simulink model "sonusimulink"  (R2015a)
settings: Solver=ode23tb  StartTime=0.0  StopTime=2  MaxStep=10e-6  RelTol=1e-3
InitFcn:
  | fs=1000;
libraries: powerlib x26, simulink x2
settings Model: Creator=KASHIF  LastModifiedBy=NITIN
settings DataIOCC: SignalLoggingSaveFormat=ModelDataLogs
settings OptimizationCC: ExpressionDepthLimit=2147483647
settings DebuggingCC: UnderspecifiedInitializationDetection=Classic  MergeDetectMultiDrivingBlocksExec=none  SolverPrmCheckMsg=warning  FcnCallInpInsideContextMsg=UseLocalSettings  StateNameClashWarn=warning
settings GRTTargetCC: CombineOutputUpdateFcns=off  GRTInterface=on

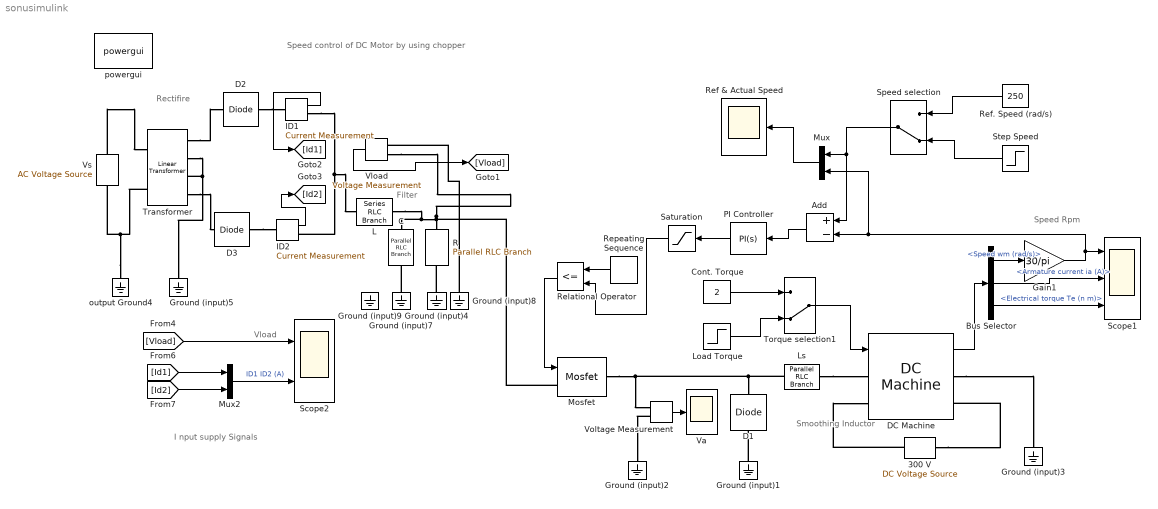
== system sonusimulink ==
  note: Speed control of DC Motor by using chopper
  note: Vload
  note: I nput supply Signals
  note: Rectifire
  note: Filter
  note: Speed Rpm
  note: Smoothing
      |  Inductor
  300 V : powerlib/Electrical Sources/DC Voltage Source  Description=source block  Amplitude=300  Measurements=None
      settings: AttributesFormatString=\n
  Add : Sum  Inputs=+-
  Bus Selector : BusSelector  OutputSignals=Speed wm (rad/s),Armature current ia (A),Electrical torque Te (n m)
  C : powerlib/Elements/Parallel RLC Branch  LConnTagsString=a  RConnTagsString=__new0  BranchType=C  Resistance=5  Inductance=1.0  SetiL0=off  InitialCurrent=0  Capacitance=500e-06  Setx0=off  InitialVoltage=0  Measurements=None
  Cont. Torque : Constant  Value=2
  D1 : powerlib/Power Electronics/Diode  Ron=0.05  Lon=0  Vf=0.7  IC=0  UseSnubber=off  Rs=Inf  Cs=0.1e-6  Measurements=off
  D2 : powerlib/Power Electronics/Diode  Ron=1e-3  Lon=0  Vf=0.7  IC=0  UseSnubber=off  Rs=1e6  Cs=inf  Measurements=off
  D3 : powerlib/Power Electronics/Diode  Ron=1e-3  Lon=0  Vf=0.7  IC=0  UseSnubber=off  Rs=1e6  Cs=inf  Measurements=off
  DC Machine : powerlib/Machines/DC Machine  PresetModel=01: 5HP 240V 1750RPM Field:300V  MechanicalLoad=Torque TL  FieldType=Wound  ShowDetailedParameters=on  MeasurementBus=off  RLa=[2.581 0.028]  RLf=[281.3 156]  Laf=0.9483  MachineConstant=Torque constant (N.m/A)  Ke=1.8  Kt=1.8  J=0.02215  Bm=0.002953  Tf=0.5161  w0=1  Ifinit=1  TsPowergui=0  TsBlock=-1
      settings: AttributesFormatString=\n
  Gain1 : Gain  Gain=30/pi
  Ground (input){1..5,7..9} (8 alike) : powerlib/Elements/Ground  LConnTagsString=a
  ID1 : powerlib/Measurements/Current Measurement  PhasorSimulation=off  OutputType=Complex  PSBequivalent=0
  ID2 : powerlib/Measurements/Current Measurement  PhasorSimulation=off  OutputType=Complex  PSBequivalent=0
  L : powerlib/Elements/Series RLC Branch  LConnTagsString=__new0  RConnTagsString=__new0  BranchType=L  Resistance=1.0  Inductance=20e-03  SetiL0=off  InitialCurrent=0  Capacitance=1.0  Setx0=off  InitialVoltage=0  Measurements=None
  Load Torque : Step  Time=1.2  Before=3  After=6  SampleTime=0
  Ls : powerlib/Elements/Parallel RLC Branch  LConnTagsString=a  RConnTagsString=__new0  BranchType=L  Resistance=1.0  Inductance=10e-03  SetiL0=off  InitialCurrent=0  Capacitance=1.0  Setx0=off  InitialVoltage=0  Measurements=None
  Mosfet : powerlib/Power Electronics/Mosfet  Ron=0.1  Lon=0  Rd=0.01  Vfd=0  IC=0  Rs=1e5  Cs=inf  Measurements=off
  Mux : Mux  Inputs=2
  Mux2 : Mux  Inputs=2
  PI Controller : simulink/Continuous/PID Controller  Controller=PI  TimeDomain=Continuous-time  SampleTime=-1  IntegratorMethod=Forward Euler  FilterMethod=Forward Euler  Form=Parallel  UseFilter=on  ControllerParametersSource=internal  P=0.001  I=0.02  D=0.0001  N=100  InitialConditionSource=internal  InitialConditionForIntegrator=0  InitialConditionForFilter=0  ExternalReset=none  LimitOutput=off  UpperSaturationLimit=inf  LowerSaturationLimit=-inf  LinearizeAsGain=off  AntiWindupMode=none  Kb=1  TrackingMode=off  Kt=1  PParamMin=[]  PParamMax=[]  IParamMin=[]  IParamMax=[]  DParamMin=[]  DParamMax=[]  NParamMin=[]  NParamMax=[]  KbParamMin=[]  KbParamMax=[]  KtParamMin=[]  KtParamMax=[]  POutMin=[]  POutMax=[]  IOutMin=[]  IOutMax=[]  DOutMin=[]  DOutMax=[]  NOutMin=[]  NOutMax=[]  KbOutMin=[]  KbOutMax=[]  KtOutMin=[]  KtOutMax=[]  IntegratorOutMin=[]  IntegratorOutMax=[]  FilterOutMin=[]  FilterOutMax=[]  SumOutMin=[]  SumOutMax=[]  SumI1OutMin=[]  SumI1OutMax=[]  SumI2OutMin=[]  SumI2OutMax=[]  SumI3OutMin=[]  SumI3OutMax=[]  SumDOutMin=[]  SumDOutMax=[]  SaturationOutMin=[]  SaturationOutMax=[]  IntegratorContinuousStateAttributes=''  IntegratorStateMustResolveToSignalObject=off  IntegratorRTWStateStorageClass=Auto  FilterContinuousStateAttributes=''  FilterStateMustResolveToSignalObject=off  FilterRTWStateStorageClass=Auto  DifferentiatorICPrevScaledInput=0  DifferentiatorOutMin=[]  DifferentiatorOutMax=[]
  R : powerlib/Elements/Parallel RLC Branch  LConnTagsString=a  RConnTagsString=__new0  BranchType=R  Resistance=10  Inductance=1.0  SetiL0=off  InitialCurrent=0  Capacitance=200e-06  Setx0=off  InitialVoltage=0  Measurements=None
  Ref & Actual Speed : Scope
      settings: TimeRange=2  YMin=2.5  YMax=800  SaveName=ScopeData2  MaxDataPoints=5000000
  Ref. Speed (rad/s) : Constant  Value=250
  Relational Operator : RelationalOperator  Operator=<=  OutDataTypeStr=boolean
  Repeating Sequence : simulink/Sources/Repeating Sequence  rep_seq_t=[0 1/2000]  rep_seq_y=[0 0.8]
  Saturation : Saturate  UpperLimit=1  LowerLimit=0
  Scope1 : Scope  NumInputPorts=3
      settings: YMin=110~0~0  YMax=800~50~15  MaxDataPoints=5000000
  Scope2 : Scope  NumInputPorts=2
      settings: ShowLegends=on  TimeRange=0.1  YMin=-1~-2.5  YMax=300~50  SaveName=ScopeData5  SampleTime=10e-6
  Speed selection : ManualSwitch  CurrentSetting=0
  "Step Speed " : Step  Time=.6  Before=200  After=400  SampleTime=0
  Torque selection1 : ManualSwitch  CurrentSetting=0
  Transformer : powerlib/Elements/Linear Transformer  UNITS=SI  NominalPower=[50 50]  winding1=[250 0 0]  winding2=[230 0 0.01]  ThreeWindings=on  winding3=[230 0 0.01]  RmLm=[Inf Inf]  Measurements=None  DataType=on
  Va : Scope
      settings: YMin=50  YMax=500  MaxDataPoints=5000000
  Vload : powerlib/Measurements/Voltage Measurement  Tag=PoWeRsYsTeMmEaSuReMeNt  PhasorSimulation=off  OutputType=Magnitude  PSBequivalent=0
  Voltage Measurement : powerlib/Measurements/Voltage Measurement  PhasorSimulation=off  OutputType=Complex  PSBequivalent=0
  Vs : powerlib/Electrical Sources/AC Voltage Source  Description=source block  Amplitude=400  Phase=0  Frequency=50  SampleTime=0  Measurements=None
      settings: AttributesFormatString=\n
  output Ground4 : powerlib/Elements/Ground  LConnTagsString=a
  powergui : powerlib/powergui  Priority=1  SimulationMode=Continuous  SolverType=Tustin/Backward Euler (TBE)  SampleTime=50e-6  frequency=60  SPID=off  DisableSnubberDevices=off  DisableRonSwitches=off  DisableVfSwitches=off  SwTol=0  DisplayEquations=off  Interpol=off  methode=off  Ts=100  FunctionMessages=off  echomessages=off  HookPort=off  EnableUseOfTLC=off  x0status=blocks  frequencyindice=0  Pbase=100e6  ErrMax=1e-4  Iterations=50  UnitsV=kV  UnitsW=MW  buscounter=0  RestoreLinks=warning  ResistiveCurrentMeasurement=off  Frange=[0:2:500]  Ylog=off  Xlog=on  ShowGrid=off  save=off  variable=ZData  structure=0  ZoomFFT=off  StartTime=0.0  cycles=1  DisplayStyle=1  fundamental=60  FreqAxis=off  MaxFrequency=1000  frequencyindicesteady=1  RmsSteady=1  display=off
  wires:
  Relational Operator/1 -> Mosfet/1
  Load Torque/1 -> Torque selection1/2
  DC Machine/1 -> Bus Selector/1
  Gain1/1 -> Scope1/1, Mux/2, Add/2
  Bus Selector/2 -> Scope1/2  "<Armature current ia (A)>"
  Bus Selector/3 -> Scope1/3  "<Electrical torque Te (n m)>"
  Voltage Measurement/1 -> Va/1
  Saturation/1 -> Relational Operator/2
  PI Controller/1 -> Saturation/1
  Add/1 -> PI Controller/1
  Mux/1 -> Ref & Actual Speed/1
  Bus Selector/1 -> Gain1/1  "<Speed wm (rad/s)>"
  Repeating Sequence/1 -> Relational Operator/1
  ID1/1 -> [Id1]
  ID2/1 -> [Id2]
  [Vload] -> Scope2/1
  Mux2/1 -> Scope2/2  "ID1 ID2 (A)"
  [Id1] -> Mux2/1
  [Id2] -> Mux2/2
  Speed selection/1 -> Add/1, Mux/1
  Ref. Speed (rad/s)/1 -> Speed selection/1
  "Step Speed "/1 -> Speed selection/2
  Cont. Torque/1 -> Torque selection1/1
  Torque selection1/1 -> DC Machine/1
  Vload/1 -> [Vload]
  connections:
  Ls/LConn1 -- Mosfet/RConn1 -- Voltage Measurement/LConn1 -- D1/RConn1
  Ls/RConn1 -- DC Machine/LConn1
  300 V/RConn1 -- DC Machine/LConn2
  300 V/LConn1 -- DC Machine/RConn2
  Ground (input)1/LConn1 -- D1/LConn1
  DC Machine/RConn1 -- Ground (input)3/LConn1
  Voltage Measurement/LConn2 -- Ground (input)2/LConn1
  output Ground4/LConn1 -- Transformer/LConn2 -- Vs/LConn1
  Vload/LConn1 -- L/RConn1 -- C/LConn1 -- Mosfet/LConn1 -- R/LConn1
  Transformer/RConn3 -- Transformer/RConn2 -- Ground (input)5/LConn1
  ID1/RConn1 -- ID2/RConn1 -- L/LConn1
  Ground (input)4/LConn1 -- R/RConn1
  Vs/RConn1 -- Transformer/LConn1
  Transformer/RConn1 -- D2/LConn1
  Ground (input)8/LConn1 -- Vload/LConn2
  Transformer/RConn4 -- D3/LConn1
  Ground (input)7/LConn1 -- C/RConn1
  D3/RConn1 -- ID2/LConn1
  D2/RConn1 -- ID1/LConn1
